simulink model "Controller"  (R2024b)
settings: Solver=ode4  StartTime=0.0  StopTime=6  FixedStep=Ts  RelTol=1e-3
values from neighbouring files (symbols this model uses):
  alpha1_val = [10; 10; 10; 5; 5; 5]    [Parameteri_mport.m]
  alpha2_val = [5; 5; 5; 2; 2; 2]    [Parameteri_mport.m]
  delta = 0.05    [Parameteri_mport.m]
  eta1 = [50; 50; 50; 20; 20; 20]    [Parameteri_mport.m]
  eta2 = [20; 20; 20; 10; 10; 10]    [Parameteri_mport.m]
  gamma1_val = 1.2    [Parameteri_mport.m]
  gamma2_val = 0.8    [Parameteri_mport.m]
  k10 = [2; 2; 2; 1; 1; 1]    [Parameteri_mport.m]
  k20 = [1; 1; 1; 0.5; 0.5; 0.5]    [Parameteri_mport.m]
  k3 = [5; 5; 5; 2; 2; 2]    [Parameteri_mport.m]
  k4 = [2; 2; 2; 1; 1; 1]    [Parameteri_mport.m]
  lambda1 = [40; 40; 40; 15; 15; 15]    [Parameteri_mport.m]
  lambda2 = [15; 15; 15; 5; 5; 5]    [Parameteri_mport.m]
undefined symbols (not defined in the file or in its folder): alpha_ar, alpha_fntsmc, beta_ar, beta_fntsmc, beta_ntsmc, eta1_val, eta2_val, gamma_ar, gamma_fntsmc, gamma_ntsmc, K0, K1_val, K2_val, K_sw, phi_val
libraries: robotmaniplib x2
settings Model: Creator=35340  LastModifiedBy=35340
settings DataIOCC: SaveFormat=Array

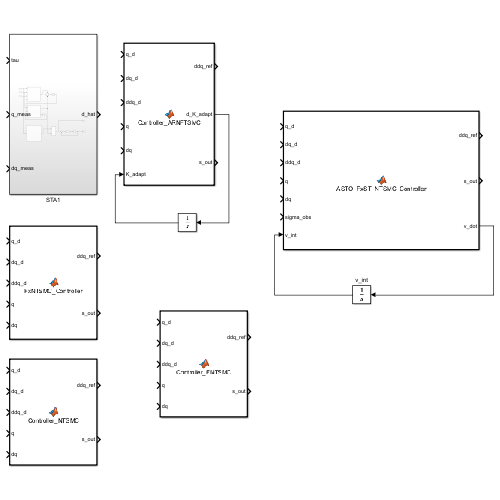
[thumbnail: Simulink's stored preview of the top-level diagram]
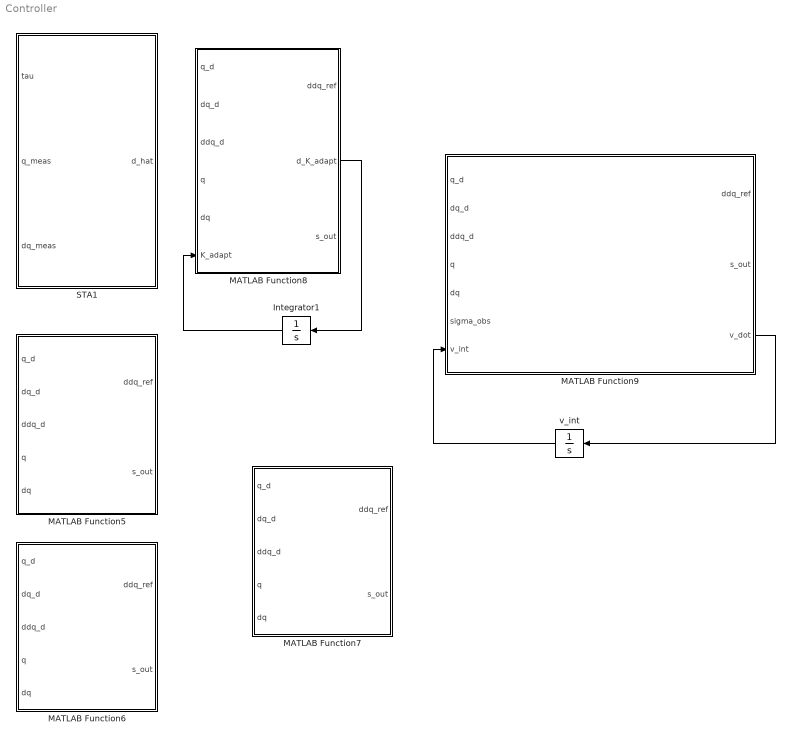
== system Controller ==
  Integrator1 : Integrator
  MATLAB Function5 : MATLAB Function  TreatAsAtomicUnit=on
  MATLAB Function6 : MATLAB Function  TreatAsAtomicUnit=on
  MATLAB Function7 : MATLAB Function  TreatAsAtomicUnit=on
  MATLAB Function8 : MATLAB Function  TreatAsAtomicUnit=on
  MATLAB Function9 : MATLAB Function  TreatAsAtomicUnit=on
  STA1 : Subsystem
  v_int : Integrator  InitialCondition=zeros(6,1)
  wires:
  MATLAB Function9/3(v_dot) -> v_int/1
  Integrator1/1 -> MATLAB Function8/6(K_adapt)
  v_int/1 -> MATLAB Function9/7(v_int)
  MATLAB Function8/2(d_K_adapt) -> Integrator1/1

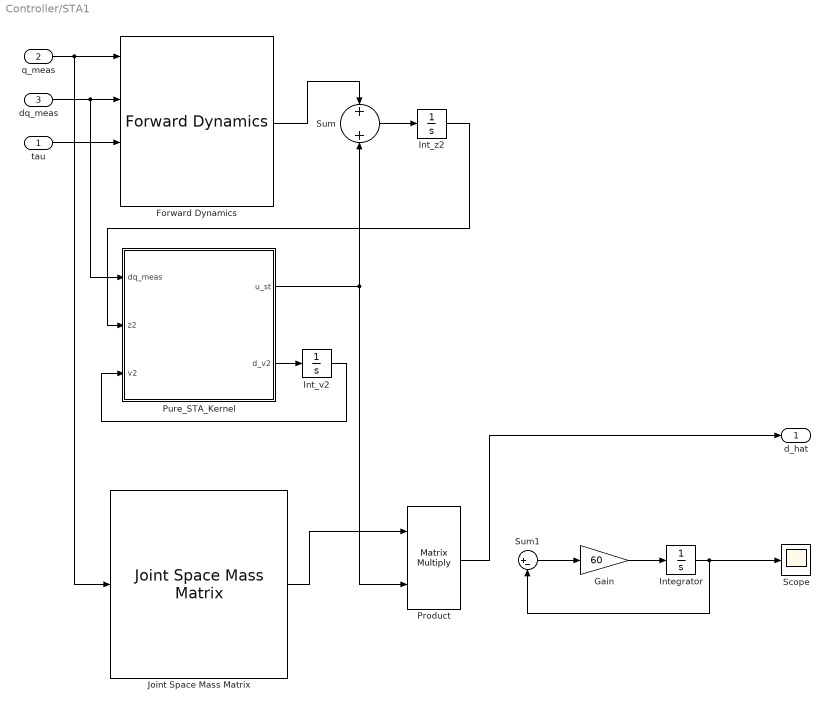
== system Controller/STA1 ==
  tau : Inport
  q_meas : Inport  Port=2
  dq_meas : Inport  Port=3
  Forward Dynamics : robotmaniplib/Forward Dynamics  RigidBodyTree=robot  SimulateUsing=Interpreted execution
  Gain : Gain  Gain=60
  Int_v2 : Integrator  InitialCondition=zeros(6,1)
  Int_z2 : Integrator  InitialCondition=zeros(6,1)
  Integrator : Integrator  InitialCondition=zeros(6,1)
  Joint Space Mass Matrix : robotmaniplib/Joint Space Mass Matrix  RigidBodyTree=robot  SimulateUsing=Interpreted execution
  Product : Product  Multiplication=Matrix(*)
  Pure_STA_Kernel : MATLAB Function  TreatAsAtomicUnit=on
  Scope : Scope
  Sum : Sum
  Sum1 : Sum  Inputs=|+-
  d_hat : Outport
  wires:
  q_meas/1 -> Forward Dynamics/1, Joint Space Mass Matrix/1
  dq_meas/1 -> Pure_STA_Kernel/1(dq_meas), Forward Dynamics/2
  tau/1 -> Forward Dynamics/3
  Forward Dynamics/1 -> Sum/1
  Sum/1 -> Int_z2/1
  Joint Space Mass Matrix/1 -> Product/1
  Gain/1 -> Integrator/1
  Integrator/1 -> Scope/1, Sum1/2
  Sum1/1 -> Gain/1
  Int_z2/1 -> Pure_STA_Kernel/2(z2)
  Int_v2/1 -> Pure_STA_Kernel/3(v2)
  Pure_STA_Kernel/2(d_v2) -> Int_v2/1
  Pure_STA_Kernel/1(u_st) -> Product/2, Sum/2
  Product/1 -> d_hat/1

== matlab function Controller/MATLAB Function9 ==
  data: q_d input; ddq_ref output; dq_d input; ddq_d input; q input; dq input; alpha1_val parameter; alpha2_val parameter; gamma1_val parameter; s_out output; v_dot output; gamma2_val parameter; k10 parameter; k20 parameter; eta1 parameter; eta2 parameter; k3 parameter; k4 parameter; sigma_obs input; v_int input
function [ddq_ref, s_out, v_dot] = ASTO_FxST_NTSMC_Controller(q_d, dq_d, ddq_d, q, dq, alpha1_val, alpha2_val, gamma1_val, gamma2_val, k10, k20, eta1, eta2, k3, k4, sigma_obs, v_int)
    % =====================================================================
    % ASTO-FxST-NTSMC: 工程极度平滑版 (消除 sign 抖振)
    % =====================================================================
    
    e = q_d - q;       
    de = dq_d - dq;    
    eps_e = 1e-4; 
    
    p = 1.5; 
    q_pow = 2.0; 
    
    % [新增核心参数]：控制器平滑边界层厚度
    % 这个值越大越平滑，0.05 是非常好的黄金点
    phi_s = 0.05; 
    
    ddq_ref = zeros(6,1);
    s = zeros(6,1);
    v_dot = zeros(6,1); 
    
    for i = 1:6
        % A. 滑模面 (保留 sign 是为了状态计算，不影响最终输出平滑度)
        term1_s = alpha1_val(i) * (abs(e(i))^gamma1_val) * sign(e(i));
        term2_s = alpha2_val(i) * (abs(e(i))^gamma2_val) * sign(e(i));
        s(i) = de(i) + term1_s + term2_s;
        
        % B. 等效控制微分项
        abs_e_safe = abs(e(i));
        if abs_e_safe < eps_e
            abs_e_safe = eps_e;
        end
        d_term1 = alpha1_val(i) * gamma1_val * (abs(e(i))^(gamma1_val - 1)) * de(i); 
        d_term2 = alpha2_val(i) * gamma2_val * (abs_e_safe^(gamma2_val - 1)) * de(i);
        
        % C. 增益联动 (因为外部传进来的是平滑误差，所以不会疯狂跳变)
        % 因为现在传进来的是平均误差，所以触发阈值要调小一点
        eps_link = 0.01;  % 从 0.05 降到 0.01
        mu = 100;         % 增加陡度，让它反应果断
        
        varpi = 1 / (1 + exp(-mu * (sigma_obs(i) - eps_link)));
        
        k1_t = k10(i) + eta1(i) * varpi;
        k2_t = k20(i) + eta2(i) * varpi;
        
        % -------------------------------------------------------------
        % D. FxST 趋近律 (!!!核心修改：全面替换 sign 为 tanh!!!)
        % -------------------------------------------------------------
        sig_s = tanh(s(i) / phi_s); % 计算平滑符号函数
        
        % 1. 比例项 (使用 sig_s 代替 sign)
        u_prop = k1_t * sqrt(abs(s(i))) * sig_s + k3(i) * (abs(s(i))^p) * sig_s;
        
        % 2. 积分项导数 (使用 sig_s 代替 sign)
        v_dot(i) = k2_t * sig_s + k4(i) * (abs(s(i))^q_pow) * sig_s;
        
        % 3. 总鲁棒项
        u_rob = u_prop + v_int(i);
                  
        % E. 合成最终参考加速度
        ddq_ref(i) = ddq_d(i) + d_term1 + d_term2 + u_rob;
        
        % 物理限幅 (保护仿真)
        limit_val = 500; 
        if ddq_ref(i) > limit_val
            ddq_ref(i) = limit_val;
        elseif ddq_ref(i) < -limit_val
            ddq_ref(i) = -limit_val;
        end
    end
    s_out = s;
end

== matlab function Controller/STA1/Pure_STA_Kernel ==
  data: dq_meas input; u_st output; z2 input; v2 input; d_v2 output; lambda1 parameter; lambda2 parameter; delta parameter
function [u_st, d_v2] = Pure_STA_Kernel(dq_meas, z2, v2, lambda1, lambda2, delta)
    % =========================================================
    % 最纯粹的传统超扭曲算法 (无任何自适应)
    % 输入: 
    %   dq_meas, z2 (用于算速度误差)
    %   v2 (积分项状态)
    %   k1, k2 (外部传入的绝对固定、巨大增益)
    % 输出:
    %   u_st (总注入项), d_v2 (积分项导数)
    % =========================================================

    % 1. 算速度误差
    sigma = dq_meas - z2;
    
    % 2. 算平滑符号函数
    sig_sigma = tanh(sigma ./ delta);
    
    % 3. 直接算注入项 (没有 omega 参与！)
    v1 = lambda1 .* sqrt(abs(sigma)) .* sig_sigma;
    d_v2 = lambda2 .* sig_sigma;
    
    % 4. 汇总
    u_st =  v1+ v2; 
end

== matlab function Controller/MATLAB Function5 ==
  data: q_d input; ddq_ref output; dq_d input; ddq_d input; q input; dq input; alpha1_val parameter; alpha2_val parameter; gamma1_val parameter; gamma2_val parameter; K1_val parameter; K2_val parameter; K0 parameter; K_sw parameter; s_out output
function [ddq_ref,s_out ] = FxNTSMC_Controller(q_d, dq_d, ddq_d, q, dq, alpha1_val, alpha2_val, gamma1_val, gamma2_val, K1_val, K2_val, K0, K_sw)
    % =====================================================================
    % FxFTSMC 复合控制器 - 绝对平滑版 (无抖振)
    % =====================================================================
    
    e = q_d - q;       
    de = dq_d - dq;    
    eps_e = 1e-4; 
    
    rho1 = 1.2; 
    rho2 = 0.8; 
    
    % 统一的平滑边界层厚度
    % 这个值越大，力矩越平滑。0.05 是非常好的黄金分割点
    phi = 0.07; 
    
    ddq_ref = zeros(6,1);
    s = zeros(6,1);
    
    for i = 1:6
        % A. 滑模面 (注意：这里保留 sign 是安全的，因为它是状态本身，不直接输出)
        term1_s = alpha1_val(i) * (abs(e(i))^gamma1_val) * sign(e(i));
        term2_s = alpha2_val(i) * (abs(e(i))^gamma2_val) * sign(e(i));
        s(i) = de(i) + term1_s + term2_s;
        
        % B. 等效控制微分项
        abs_e_safe = abs(e(i));
        if abs_e_safe < eps_e
            abs_e_safe = eps_e;
        end
        d_term1 = alpha1_val(i) * gamma1_val * (abs(e(i))^(gamma1_val - 1)) * de(i); 
        d_term2 = alpha2_val(i) * gamma2_val * (abs_e_safe^(gamma2_val - 1)) * de(i);
        
        % -------------------------------------------------------------
        % C. 复合趋近律 (彻底替换为 tanh，完全消灭不连续切换)
        % -------------------------------------------------------------
        robust_term = K1_val(i) * (abs(s(i))^rho1) * tanh(s(i)/phi) + ... % 远端平滑
                      K2_val(i) * (abs(s(i))^rho2) * tanh(s(i)/phi) + ... % 近端平滑
                      K0(i) * s(i) + ...                              % 线性项
                      K_sw(i) * tanh(s(i)/phi);                       % 鲁棒项
                  
        % D. 合成最终参考加速度
        ddq_ref(i) = ddq_d(i) + d_term1 + d_term2 + robust_term;
        
        % 物理限幅 (稍微缩紧一点，防止起步瞬间力矩过大)
        limit_val = 500; 
        if ddq_ref(i) > limit_val
            ddq_ref(i) = limit_val;
        elseif ddq_ref(i) < -limit_val
            ddq_ref(i) = -limit_val;
        end
    end
    s_out = s;
end

== matlab function Controller/MATLAB Function6 ==
  data: q_d input; ddq_ref output; dq_d input; ddq_d input; q input; dq input; beta_ntsmc parameter; gamma_ntsmc parameter; K1_val parameter; K2_val parameter; phi_val parameter; s_out output
function [ddq_ref, s_out] = Controller_NTSMC(q_d, dq_d, ddq_d, q, dq, beta_ntsmc, gamma_ntsmc, K1_val, K2_val, phi_val)
    e = q_d - q;       
    de = dq_d - dq;    
    eps_e = 1e-4; 
    
    ddq_ref = zeros(6,1);
    s = zeros(6,1); % 必须在这里初始化为 6x1 向量！
    
    for i = 1:6
        % 注意这里必须是 s(i)
        s(i) = e(i) + beta_ntsmc(i) * (abs(de(i))^gamma_ntsmc) * sign(de(i));
        
        abs_de = abs(de(i));
        if abs_de < eps_e, abs_de = eps_e; end 
        Lambda = beta_ntsmc(i) * gamma_ntsmc * (abs_de^(gamma_ntsmc - 1));
        
        robust = K1_val(i)*s(i) + K2_val(i)*tanh(s(i)/phi_val);
        ddq_ref(i) = ddq_d(i) + (de(i) + robust) / Lambda;
        
        if ddq_ref(i) > 200, ddq_ref(i) = 200; elseif ddq_ref(i) < -200, ddq_ref(i) = -200; end
    end
    s_out = s; % 最终输出 6x1 向量
end

== matlab function Controller/MATLAB Function7 ==
  data: q_d input; ddq_ref output; dq_d input; ddq_d input; q input; dq input; alpha_fntsmc parameter; beta_fntsmc parameter; gamma_fntsmc parameter; K1_val parameter; K2_val parameter; phi_val parameter; s_out output
function [ddq_ref, s_out] = Controller_FNTSMC(q_d, dq_d, ddq_d, q, dq, alpha_fntsmc, beta_fntsmc, gamma_fntsmc, K1_val, K2_val, phi_val)
    e = q_d - q;       
    de = dq_d - dq;    
    eps_e = 1e-4; 
    
    ddq_ref = zeros(6,1);
    s = zeros(6,1); % 初始化
    
    for i = 1:6
        % 注意这里必须是 s(i)
        s(i) = de(i) + alpha_fntsmc(i)*e(i) + beta_fntsmc(i)*(abs(e(i))^gamma_fntsmc)*sign(e(i));
        
        abs_e = abs(e(i));
        if abs_e < eps_e, abs_e = eps_e; end 
        
        d_term = alpha_fntsmc(i)*de(i) + beta_fntsmc(i)*gamma_fntsmc*(abs_e^(gamma_fntsmc-1))*de(i);
        robust = K1_val(i)*s(i) + K2_val(i)*tanh(s(i)/phi_val);
        
        ddq_ref(i) = ddq_d(i) + d_term + robust;
        
        if ddq_ref(i) > 200, ddq_ref(i) = 200; elseif ddq_ref(i) < -200, ddq_ref(i) = -200; end
    end
    s_out = s; % 输出
end

== matlab function Controller/MATLAB Function8 ==
  data: q_d input; ddq_ref output; dq_d input; ddq_d input; q input; dq input; K_adapt input; alpha_ar parameter; beta_ar parameter; gamma_ar parameter; eta1_val parameter; eta2_val parameter; phi_val parameter; d_K_adapt output; s_out output
function [ddq_ref, d_K_adapt, s_out] = Controller_ARNFTSMC(q_d, dq_d, ddq_d, q, dq, K_adapt, alpha_ar, beta_ar, gamma_ar, eta1_val, eta2_val, phi_val)
    e = q_d - q;       
    de = dq_d - dq;    
    eps_e = 1e-4; 
    
    ddq_ref = zeros(6,1);
    d_K_adapt = zeros(6,1);
    s = zeros(6,1); % 初始化
    
    for i = 1:6
        % 注意这里必须是 s(i)
        s(i) = de(i) + alpha_ar(i)*e(i) + beta_ar(i)*(abs(e(i))^gamma_ar)*sign(e(i));
        
        abs_e = abs(e(i));
        if abs_e < eps_e, abs_e = eps_e; end 
        d_term = alpha_ar(i)*de(i) + beta_ar(i)*gamma_ar*(abs_e^(gamma_ar-1))*de(i);
        
        robust = K_adapt(i) * tanh(s(i) / phi_val);
        
        d_K_adapt(i) = eta1_val(i) * abs(s(i)) - eta2_val(i) * K_adapt(i);
        
        ddq_ref(i) = ddq_d(i) + d_term + robust;
        
        if ddq_ref(i) > 200, ddq_ref(i) = 200; elseif ddq_ref(i) < -200, ddq_ref(i) = -200; end
    end
    s_out = s; % 输出
end
